simulink model "PMSM_VC2"  (Simulink 7.5)
settings: Solver=ode45  StartTime=0.0  StopTime=0.5  RelTol=1e-3
undefined symbols (not defined in the file): DiscIntNeverNeededParam
libraries: powerlib x4, simulink x1
settings Model: Creator=LZ  LastModifiedBy=LZ  SimulationMode=accelerator  CovModelRefEnable=off
settings DataIOCC: LimitDataPoints=off  SaveFormat=StructureWithTime
settings OptimizationCC: ExpressionDepthLimit=128
settings DebuggingCC: UnderspecifiedInitializationDetection=Simplified  MergeDetectMultiDrivingBlocksExec=error  SolverPrmCheckMsg=none  FcnCallInpInsideContextMsg=Enable All  StateNameClashWarn=none
settings HardwareCC: ProdIntDivRoundTo=Zero  ProdEndianess=LittleEndian  ProdHWDeviceType=Specified
settings CodeAppCC: CustomSymbolStrType=$N$R$M_T
settings GRTTargetCC: TargetFunctionLibrary=C89/C90 (ANSI)

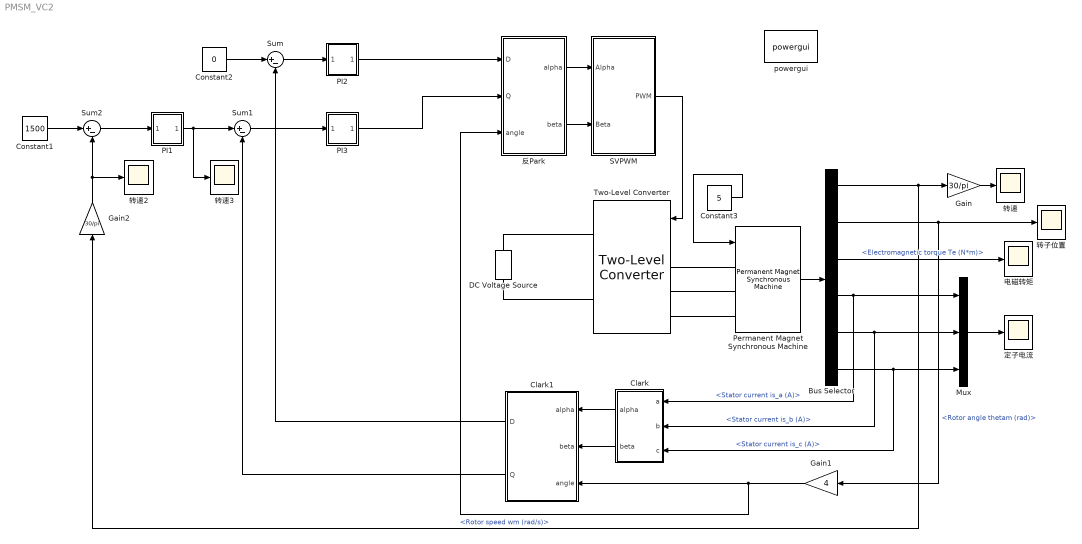
== system PMSM_VC2 ==
  Bus Selector : BusSelector  OutputSignals=Rotor speed wm (rad/s),Rotor angle thetam (rad),Electromagnetic torque Te (N*m),Stator current is_a (A),Stator current is_b (A),Stator current is_c (A)
  Clark : Subsystem
  Clark1 : Subsystem
  Constant1 : Constant  Value=1500
  Constant2 : Constant  Value=0
  Constant3 : Constant  Value=5
  DC Voltage Source : powerlib/Electrical Sources/DC Voltage Source  Amplitude=560  Measurements=None
  Gain : Gain  Gain=30/pi
  Gain1 : Gain  Gain=4
  Gain2 : Gain  Gain=30/pi
  Mux : Mux  Inputs=3
  PI1 : Subsystem  mask{Kp=0.5, Ki=80, Par_limits=[30 -30], Init=0, Ts=1e-6}
      mask prompts: Kp "Proportional gain(Kp)"; Ki "Integral gain(Ki)"; Par_limits "Output limits:[Upper Lower]"; Init "Output initial value"; Ts "Sample time"
      mask init:
      | Upperlimit = Par_limits(1);
      | Lowerlimit = Par_limits(2);
      mask Display: disp('PI')
  PI2 : Subsystem  mask{Kp=4, Ki=60, Par_limits=[150 -150], Init=0, Ts=1e-6}
      mask prompts: Kp "Proportional gain(Kp)"; Ki "Integral gain(Ki)"; Par_limits "Output limits:[Upper Lower]"; Init "Output initial value"; Ts "Sample time"
      mask init:
      | Upperlimit = Par_limits(1);
      | Lowerlimit = Par_limits(2);
      mask Display: disp('PI')
  PI3 : Subsystem  mask{Kp=4, Ki=60, Par_limits=[150 -150], Init=0, Ts=1e-6}
      mask prompts: Kp "Proportional gain(Kp)"; Ki "Integral gain(Ki)"; Par_limits "Output limits:[Upper Lower]"; Init "Output initial value"; Ts "Sample time"
      mask init:
      | Upperlimit = Par_limits(1);
      | Lowerlimit = Par_limits(2);
      mask Display: disp('PI')
  Permanent Magnet Synchronous Machine : powerlib/Machines/Permanent Magnet Synchronous Machine  NbPhases=3  FluxDistribution=Sinusoidal  RotorType=Round  MechanicalLoad=Torque Tm  PresetModel="11:  26.13 Nm 560 Vdc 3000 RPM - 27.3 Nm"  ShowDetailedParameters=on  MeasurementBus=off  Resistance=0.11  Inductance=8.5e-3  dqInductances=[8.5e-3,8.5e-3]  La=0.00097  MachineConstant=Flux linkage established by magnets (V.s)  Flux=0.1119  VoltageCst=81.1857  TorqueCst=0.6714  Flat=120  Mechanical=[0.0016 0.0002024 4 0]  PolePairs=4  InitialConditions=[0,0, 0,0]  InitialConditions5ph=[0 0 0 0 0 0]  TsPowergui=0  TsBlock=-1  RefAngle=Aligned with phase A axis (original Park)
  SVPWM : Subsystem
  Sum : Sum  Inputs=|+-
  Sum1 : Sum  Inputs=|+-
  Sum2 : Sum  Inputs=|+-
  Two-Level Converter : powerlib/Power Electronics/Two-Level Converter  ModelType=Switching devices  Ron=1e-3  Rs=1e6  Cs=inf  Vforward=[0,0]  Ron_Diode=1e-3  Rs_Diode=1e6  Cs_Diode=inf  Vf_Diode=1e-3  Rs_CurrentSource=inf
  powergui : powerlib/powergui  Priority=1  SimulationMode=Discrete  SolverType=Tustin/Backward Euler (TBE)  SampleTime=1e-6  frequency=60  SPID=off  DisableSnubberDevices=off  DisableRonSwitches=off  DisableVfSwitches=off  SwTol=0  DisplayEquations=off  Interpol=off  ExternalGateDelay=off  methode=off  Ts=10  FunctionMessages=off  echomessages=off  HookPort=off  EnableUseOfTLC=off  x0status=blocks  frequencyindice=0  Pbase=100e6  ErrMax=1e-4  Iterations=50  UnitsV=kV  UnitsW=MW  buscounter=0  RestoreLinks=warning  ResistiveCurrentMeasurement=off  Frange=[0:2:500]  Ylog=off  Xlog=on  ShowGrid=off  save=off  variable=ZData  structure=0  ZoomFFT=off  StartTime=0.0  cycles=1  DisplayStyle=1  fundamental=60  FreqAxis=off  MaxFrequency=1000  frequencyindicesteady=1  RmsSteady=1  display=off
  反Park : Subsystem
  定子电流 : Scope
      settings: TimeRange=auto  MaxDataPoints=5000  SaveToWorkspace=off  SaveName=ScopeData3  YMin=-49.88136  YMax=50.05576  SampleTime=-1  DataFormat=Array
  电磁转矩 : Scope
      settings: TimeRange=auto  MaxDataPoints=5000  SaveToWorkspace=off  SaveName=ScopeData2  YMin=-3.8739  YMax=34.86513  SampleTime=-1  DataFormat=Array
  转子位置 : Scope
      settings: TimeRange=auto  MaxDataPoints=5000  SaveToWorkspace=off  YMin=-9.57744  YMax=86.1955  SampleTime=-1
  转速 : Scope
      settings: TimeRange=auto  MaxDataPoints=5000  SaveToWorkspace=off  SaveName=ScopeData  YMin=-196.87171  YMax=1710.56254  SampleTime=-1
  转速2 : Scope
      settings: TimeRange=auto  MaxDataPoints=5000  SaveToWorkspace=off  SaveName=ScopeData4  YMin=-196.87171  YMax=1710.56254  SampleTime=-1
  转速3 : Scope
      settings: TimeRange=auto  MaxDataPoints=5000  SaveToWorkspace=off  SaveName=ScopeData7  YMin=-21.21411  YMax=35.69046  SampleTime=-1
  wires:
  Permanent Magnet Synchronous Machine/1 -> Bus Selector/1
  Bus Selector/1 -> Gain2/1, Gain/1  "<Rotor speed wm (rad/s)>"
  Gain/1 -> 转速/1
  Bus Selector/2 -> Gain1/1, 转子位置/1  "<Rotor angle thetam (rad)>"
  Bus Selector/3 -> 电磁转矩/1  "<Electromagnetic torque Te (N*m)>"
  Bus Selector/6 -> Clark/3(c), Mux/3  "<Stator current is_c (A)>"
  Bus Selector/5 -> Clark/2(b), Mux/2  "<Stator current is_b (A)>"
  Bus Selector/4 -> Clark/1(a), Mux/1  "<Stator current is_a (A)>"
  Mux/1 -> 定子电流/1
  SVPWM/1(PWM) -> Two-Level Converter/1
  Gain1/1 -> Clark1/3(angle), 反Park/3(angle)
  Clark1/2(Q) -> Sum1/2
  Clark1/1(D) -> Sum/2
  Sum1/1 -> PI3/1(Err)
  Sum/1 -> PI2/1(Err)
  PI1/1(Out1) -> 转速3/1, Sum1/1
  PI2/1(Out1) -> 反Park/1(D)
  PI3/1(Out1) -> 反Park/2(Q)
  Gain2/1 -> 转速2/1, Sum2/2
  Sum2/1 -> PI1/1(Err)
  Constant1/1 -> Sum2/1
  Constant2/1 -> Sum/1
  Clark/1(alpha) -> Clark1/1(alpha)
  Clark/2(beta) -> Clark1/2(beta)
  反Park/1(alpha) -> SVPWM/1(Alpha)
  反Park/2(beta) -> SVPWM/2(Beta)
  Constant3/1 -> Permanent Magnet Synchronous Machine/1
  connections:
  DC Voltage Source/LConn1 -- Two-Level Converter/RConn2
  Two-Level Converter/LConn1 -- Permanent Magnet Synchronous Machine/LConn1
  DC Voltage Source/RConn1 -- Two-Level Converter/RConn1
  Two-Level Converter/LConn3 -- Permanent Magnet Synchronous Machine/LConn3
  Two-Level Converter/LConn2 -- Permanent Magnet Synchronous Machine/LConn2

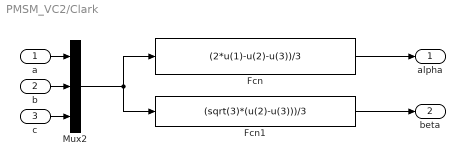
== system PMSM_VC2/Clark ==
  a : Inport
  b : Inport  Port=2
  c : Inport  Port=3
  Fcn : Fcn  Expr=(2*u(1)-u(2)-u(3))/3
  Fcn1 : Fcn  Expr=(sqrt(3)*(u(2)-u(3)))/3
  Mux2 : Mux  Inputs=3
  alpha : Outport
  beta : Outport  Port=2
  wires:
  Mux2/1 -> Fcn/1, Fcn1/1
  Fcn/1 -> alpha/1
  Fcn1/1 -> beta/1
  c/1 -> Mux2/3
  a/1 -> Mux2/1
  b/1 -> Mux2/2

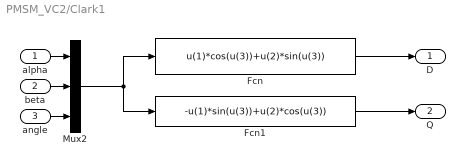
== system PMSM_VC2/Clark1 ==
  alpha : Inport
  beta : Inport  Port=2
  angle : Inport  Port=3
  Fcn : Fcn  Expr=u(1)*cos(u(3))+u(2)*sin(u(3))
  Fcn1 : Fcn  Expr=-u(1)*sin(u(3))+u(2)*cos(u(3))
  Mux2 : Mux  Inputs=3
  D : Outport
  Q : Outport  Port=2
  wires:
  beta/1 -> Mux2/2
  alpha/1 -> Mux2/1
  angle/1 -> Mux2/3
  Fcn1/1 -> Q/1
  Fcn/1 -> D/1
  Mux2/1 -> Fcn1/1, Fcn/1

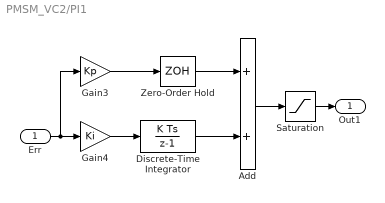
== system PMSM_VC2/PI1 ==
  Err : Inport
  Add : Sum
  Discrete-Time Integrator : DiscreteIntegrator  InitialCondition=Init  SampleTime=Ts  LimitOutput=on  UpperSaturationLimit=Upperlimit  LowerSaturationLimit=Lowerlimit  ICPrevOutput=DiscIntNeverNeededParam  ICPrevScaledInput=DiscIntNeverNeededParam
  Gain3 : Gain  Gain=Kp
  Gain4 : Gain  Gain=Ki
  Saturation : Saturate  UpperLimit=Upperlimit  LowerLimit=Lowerlimit
  Zero-Order Hold : ZeroOrderHold  SampleTime=Ts
  Out1 : Outport
  wires:
  Zero-Order Hold/1 -> Add/1
  Gain4/1 -> Discrete-Time Integrator/1
  Saturation/1 -> Out1/1
  Err/1 -> Gain4/1, Gain3/1
  Add/1 -> Saturation/1
  Discrete-Time Integrator/1 -> Add/2
  Gain3/1 -> Zero-Order Hold/1

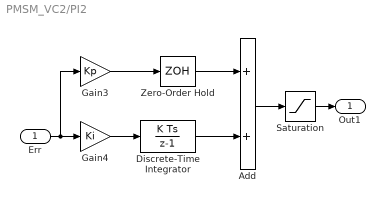
== system PMSM_VC2/PI2 ==
  Err : Inport
  Add : Sum
  Discrete-Time Integrator : DiscreteIntegrator  InitialCondition=Init  SampleTime=Ts  LimitOutput=on  UpperSaturationLimit=Upperlimit  LowerSaturationLimit=Lowerlimit  ICPrevOutput=DiscIntNeverNeededParam  ICPrevScaledInput=DiscIntNeverNeededParam
  Gain3 : Gain  Gain=Kp
  Gain4 : Gain  Gain=Ki
  Saturation : Saturate  UpperLimit=Upperlimit  LowerLimit=Lowerlimit
  Zero-Order Hold : ZeroOrderHold  SampleTime=Ts
  Out1 : Outport
  wires:
  Gain3/1 -> Zero-Order Hold/1
  Discrete-Time Integrator/1 -> Add/2
  Add/1 -> Saturation/1
  Err/1 -> Gain3/1, Gain4/1
  Saturation/1 -> Out1/1
  Gain4/1 -> Discrete-Time Integrator/1
  Zero-Order Hold/1 -> Add/1

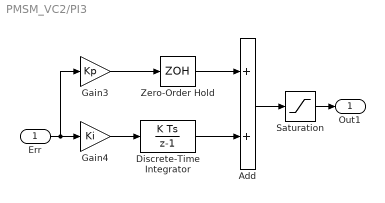
== system PMSM_VC2/PI3 ==
  Err : Inport
  Add : Sum
  Discrete-Time Integrator : DiscreteIntegrator  InitialCondition=Init  SampleTime=Ts  LimitOutput=on  UpperSaturationLimit=Upperlimit  LowerSaturationLimit=Lowerlimit  ICPrevOutput=DiscIntNeverNeededParam  ICPrevScaledInput=DiscIntNeverNeededParam
  Gain3 : Gain  Gain=Kp
  Gain4 : Gain  Gain=Ki
  Saturation : Saturate  UpperLimit=Upperlimit  LowerLimit=Lowerlimit
  Zero-Order Hold : ZeroOrderHold  SampleTime=Ts
  Out1 : Outport
  wires:
  Zero-Order Hold/1 -> Add/1
  Gain4/1 -> Discrete-Time Integrator/1
  Saturation/1 -> Out1/1
  Err/1 -> Gain4/1, Gain3/1
  Add/1 -> Saturation/1
  Discrete-Time Integrator/1 -> Add/2
  Gain3/1 -> Zero-Order Hold/1

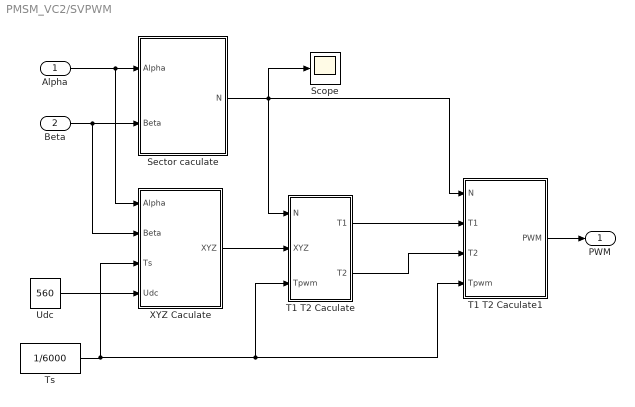
== system PMSM_VC2/SVPWM ==
  Alpha : Inport
  Beta : Inport  Port=2
  Scope : Scope
      settings: TimeRange=auto  MaxDataPoints=5000  SaveToWorkspace=off  SaveName=ScopeData6  YMin=0.375  YMax=6.625  SampleTime=-1
  Sector caculate : Subsystem
  T1 T2 Caculate : Subsystem
  T1 T2 Caculate1 : Subsystem
  Ts : Constant  Value=1/6000
  Udc : Constant  Value=560
  XYZ Caculate : Subsystem
  PWM : Outport
  wires:
  Alpha/1 -> XYZ Caculate/1(Alpha), Sector caculate/1(Alpha)
  Beta/1 -> XYZ Caculate/2(Beta), Sector caculate/2(Beta)
  Sector caculate/1(N) -> Scope/1, T1 T2 Caculate/1(N), T1 T2 Caculate1/1(N)
  T1 T2 Caculate1/1(PWM) -> PWM/1
  T1 T2 Caculate/1(T1) -> T1 T2 Caculate1/2(T1)
  T1 T2 Caculate/2(T2) -> T1 T2 Caculate1/3(T2)
  XYZ Caculate/1(XYZ) -> T1 T2 Caculate/2(XYZ)
  Ts/1 -> T1 T2 Caculate1/4(Tpwm), T1 T2 Caculate/3(Tpwm), XYZ Caculate/3(Ts)
  Udc/1 -> XYZ Caculate/4(Udc)

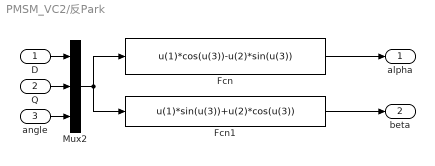
== system PMSM_VC2/反Park ==
  D : Inport
  Q : Inport  Port=2
  angle : Inport  Port=3
  Fcn : Fcn  Expr=u(1)*cos(u(3))-u(2)*sin(u(3))
  Fcn1 : Fcn  Expr=u(1)*sin(u(3))+u(2)*cos(u(3))
  Mux2 : Mux  Inputs=3
  alpha : Outport
  beta : Outport  Port=2
  wires:
  Q/1 -> Mux2/2
  D/1 -> Mux2/1
  angle/1 -> Mux2/3
  Fcn1/1 -> beta/1
  Fcn/1 -> alpha/1
  Mux2/1 -> Fcn1/1, Fcn/1

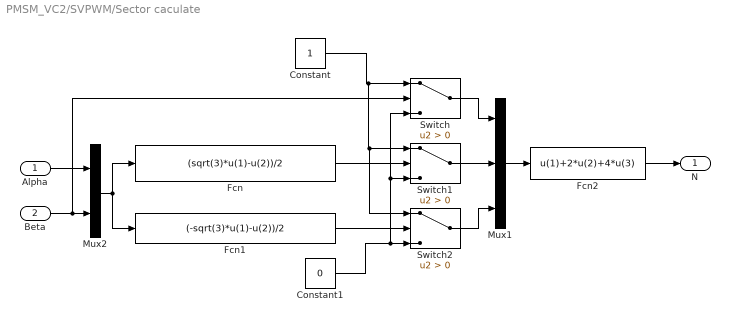
== system PMSM_VC2/SVPWM/Sector caculate ==
  Alpha : Inport
  Beta : Inport  Port=2
  Constant : Constant
  Constant1 : Constant  Value=0
  Fcn : Fcn  Expr=(sqrt(3)*u(1)-u(2))/2
  Fcn1 : Fcn  Expr=(-sqrt(3)*u(1)-u(2))/2
  Fcn2 : Fcn  Expr=u(1)+2*u(2)+4*u(3)
  Mux1 : Mux  Inputs=3
  Mux2 : Mux  Inputs=2
  Switch : Switch  Criteria=u2 > Threshold
  Switch1 : Switch  Criteria=u2 > Threshold
  Switch2 : Switch  Criteria=u2 > Threshold
  N : Outport
  wires:
  Switch/1 -> Mux1/1
  Switch1/1 -> Mux1/2
  Fcn/1 -> Switch1/2
  Mux2/1 -> Fcn/1, Fcn1/1
  Fcn1/1 -> Switch2/2
  Alpha/1 -> Mux2/1
  Beta/1 -> Switch/2, Mux2/2
  Fcn2/1 -> N/1
  Constant/1 -> Switch2/1, Switch1/1, Switch/1
  Switch2/1 -> Mux1/3
  Constant1/1 -> Switch1/3, Switch/3, Switch2/3
  Mux1/1 -> Fcn2/1

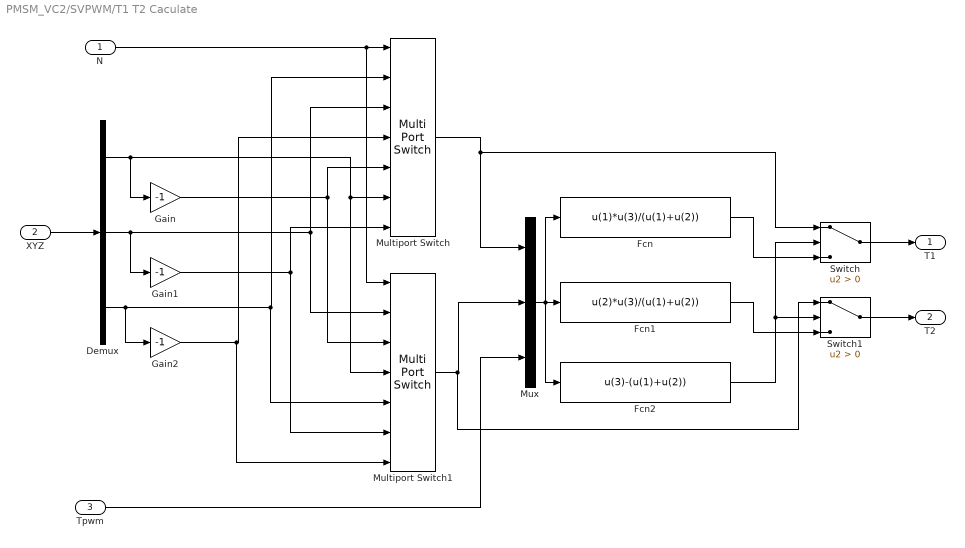
== system PMSM_VC2/SVPWM/T1 T2 Caculate ==
  N : Inport
  XYZ : Inport  Port=2
  Tpwm : Inport  Port=3
  Demux : Demux  Outputs=3
  Fcn : Fcn  Expr=u(1)*u(3)/(u(1)+u(2))
  Fcn1 : Fcn  Expr=u(2)*u(3)/(u(1)+u(2))
  Fcn2 : Fcn  Expr=u(3)-(u(1)+u(2))
  Gain : Gain  Gain=-1
  Gain1 : Gain  Gain=-1
  Gain2 : Gain  Gain=-1
  Multiport Switch : MultiPortSwitch  Inputs=6
  Multiport Switch1 : MultiPortSwitch  Inputs=6
  Mux : Mux  Inputs=3
  Switch : Switch  Criteria=u2 > Threshold
  Switch1 : Switch  Criteria=u2 > Threshold
  T1 : Outport
  T2 : Outport  Port=2
  wires:
  XYZ/1 -> Demux/1
  N/1 -> Multiport Switch1/1, Multiport Switch/1
  Demux/1 -> Gain/1, Multiport Switch1/4, Multiport Switch/6
  Gain/1 -> Multiport Switch/5, Multiport Switch1/3
  Demux/2 -> Gain1/1, Multiport Switch1/2, Multiport Switch/3
  Gain1/1 -> Multiport Switch1/6, Multiport Switch/7
  Demux/3 -> Gain2/1, Multiport Switch1/5, Multiport Switch/2
  Gain2/1 -> Multiport Switch1/7, Multiport Switch/4
  Switch/1 -> T1/1
  Switch1/1 -> T2/1
  Mux/1 -> Fcn2/1, Fcn/1, Fcn1/1
  Tpwm/1 -> Mux/3
  Multiport Switch1/1 -> Switch1/1, Mux/2
  Multiport Switch/1 -> Switch/1, Mux/1
  Fcn2/1 -> Switch/2, Switch1/2
  Fcn/1 -> Switch/3
  Fcn1/1 -> Switch1/3

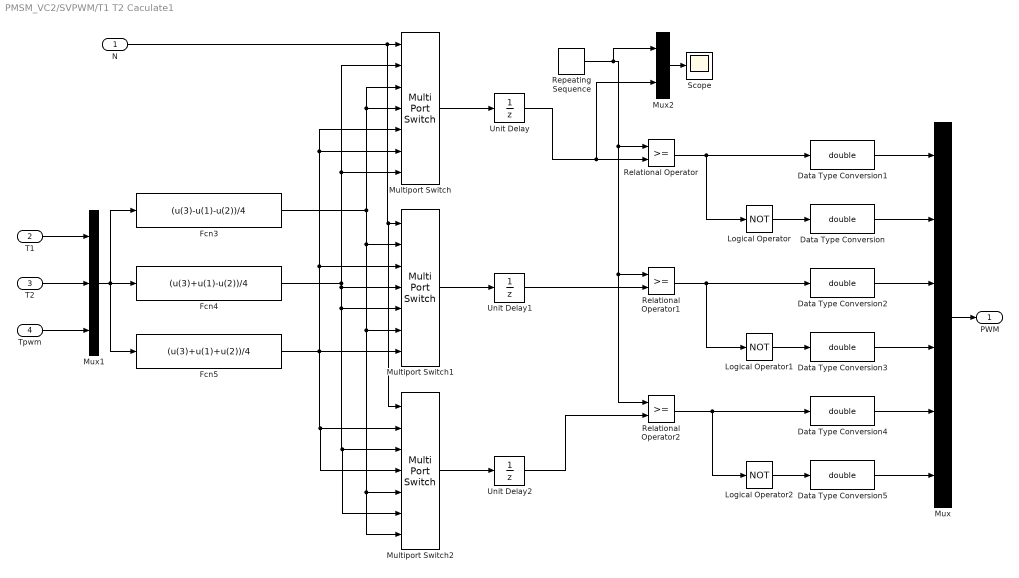
== system PMSM_VC2/SVPWM/T1 T2 Caculate1 ==
  N : Inport
  T1 : Inport  Port=2
  T2 : Inport  Port=3
  Tpwm : Inport  Port=4
  Data Type Conversion{,1..5} (6 alike) : DataTypeConversion  OutDataTypeStr=double  OutDataTypeMode=double
  Fcn3 : Fcn  Expr=(u(3)-u(1)-u(2))/4
  Fcn4 : Fcn  Expr=(u(3)+u(1)-u(2))/4
  Fcn5 : Fcn  Expr=(u(3)+u(1)+u(2))/4
  Logical Operator : Logic  Operator=NOT  AllPortsSameDT=off  OutDataTypeStr=boolean  OutDataTypeMode=boolean
  Logical Operator1 : Logic  Operator=NOT  AllPortsSameDT=off  OutDataTypeStr=boolean  OutDataTypeMode=boolean
  Logical Operator2 : Logic  Operator=NOT  AllPortsSameDT=off  OutDataTypeStr=boolean  OutDataTypeMode=boolean
  Multiport Switch : MultiPortSwitch  Inputs=6
  Multiport Switch1 : MultiPortSwitch  Inputs=6
  Multiport Switch2 : MultiPortSwitch  Inputs=6
  Mux : Mux  Inputs=6
  Mux1 : Mux  Inputs=3
  Mux2 : Mux  Inputs=2
  Relational Operator : RelationalOperator  OutDataTypeStr=boolean  LogicOutDataTypeMode=boolean
  Relational Operator1 : RelationalOperator  OutDataTypeStr=boolean  LogicOutDataTypeMode=boolean
  Relational Operator2 : RelationalOperator  OutDataTypeStr=boolean  LogicOutDataTypeMode=boolean
  Repeating Sequence : simulink/Sources/Repeating Sequence  rep_seq_t=[0 1/12000 1/6000]  rep_seq_y=[0 1/12000 0]
  Scope : Scope
      settings: TimeRange=auto  MaxDataPoints=5000  SaveToWorkspace=off  SaveName=ScopeData5  YMin=-0.00001  YMax=0.00009  SampleTime=-1
  Unit Delay : UnitDelay  SampleTime=1/6000
  Unit Delay1 : UnitDelay  SampleTime=1/6000
  Unit Delay2 : UnitDelay  SampleTime=1/6000
  PWM : Outport
  wires:
  T1/1 -> Mux1/1
  T2/1 -> Mux1/2
  Tpwm/1 -> Mux1/3
  Mux1/1 -> Fcn5/1, Fcn3/1, Fcn4/1
  N/1 -> Multiport Switch2/1, Multiport Switch1/1, Multiport Switch/1
  Fcn3/1 -> Multiport Switch2/7, Multiport Switch2/5, Multiport Switch1/6, Multiport Switch1/2, Multiport Switch/3, Multiport Switch/4
  Fcn4/1 -> Multiport Switch2/6, Multiport Switch2/3, Multiport Switch1/5, Multiport Switch1/4, Multiport Switch/7, Multiport Switch/2
  Fcn5/1 -> Multiport Switch2/4, Multiport Switch2/2, Multiport Switch1/7, Multiport Switch/6, Multiport Switch/5, Multiport Switch1/3
  Logical Operator2/1 -> Data Type Conversion5/1
  Data Type Conversion5/1 -> Mux/6
  Repeating Sequence/1 -> Mux2/1, Relational Operator2/1, Relational Operator1/1, Relational Operator/1
  Relational Operator/1 -> Logical Operator/1, Data Type Conversion1/1
  Data Type Conversion1/1 -> Mux/1
  Logical Operator/1 -> Data Type Conversion/1
  Data Type Conversion/1 -> Mux/2
  Relational Operator1/1 -> Logical Operator1/1, Data Type Conversion2/1
  Logical Operator1/1 -> Data Type Conversion3/1
  Data Type Conversion2/1 -> Mux/3
  Data Type Conversion3/1 -> Mux/4
  Data Type Conversion4/1 -> Mux/5
  Relational Operator2/1 -> Logical Operator2/1, Data Type Conversion4/1
  Multiport Switch2/1 -> Unit Delay2/1
  Multiport Switch1/1 -> Unit Delay1/1
  Multiport Switch/1 -> Unit Delay/1
  Mux2/1 -> Scope/1
  Mux/1 -> PWM/1
  Unit Delay/1 -> Mux2/2, Relational Operator/2
  Unit Delay1/1 -> Relational Operator1/2
  Unit Delay2/1 -> Relational Operator2/2

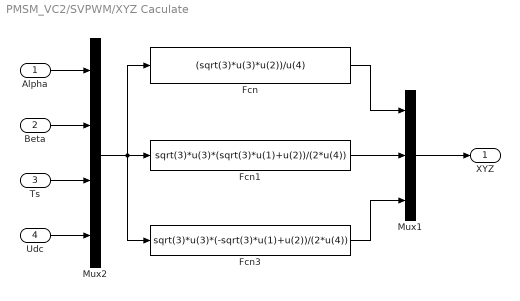
== system PMSM_VC2/SVPWM/XYZ Caculate ==
  Alpha : Inport
  Beta : Inport  Port=2
  Ts : Inport  Port=3
  Udc : Inport  Port=4
  Fcn : Fcn  Expr=(sqrt(3)*u(3)*u(2))/u(4)
  Fcn1 : Fcn  Expr=sqrt(3)*u(3)*(sqrt(3)*u(1)+u(2))/(2*u(4))
  Fcn3 : Fcn  Expr=sqrt(3)*u(3)*(-sqrt(3)*u(1)+u(2))/(2*u(4))
  Mux1 : Mux  Inputs=3
  Mux2 : Mux
  XYZ : Outport
  wires:
  Mux1/1 -> XYZ/1
  Beta/1 -> Mux2/2
  Alpha/1 -> Mux2/1
  Mux2/1 -> Fcn3/1, Fcn/1, Fcn1/1
  Fcn/1 -> Mux1/1
  Fcn1/1 -> Mux1/2
  Fcn3/1 -> Mux1/3
  Ts/1 -> Mux2/3
  Udc/1 -> Mux2/4
